simulink model "Aries_2"  (R2026a)
settings: Solver=VariableStepAuto  StopTime=0.05
undefined symbols (not defined in the file): physconst
libraries: phasedtxrxlib x4, phasedenvlib x3, phaseddetectlib x2, phasedwavlib x1, phasedbflib x1
settings Model: Creator=Anunnya  LastModifiedBy=Anunnya

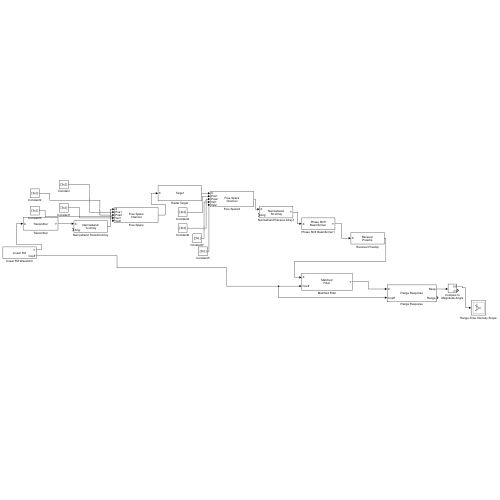
[thumbnail: Simulink's stored preview of the top-level diagram]
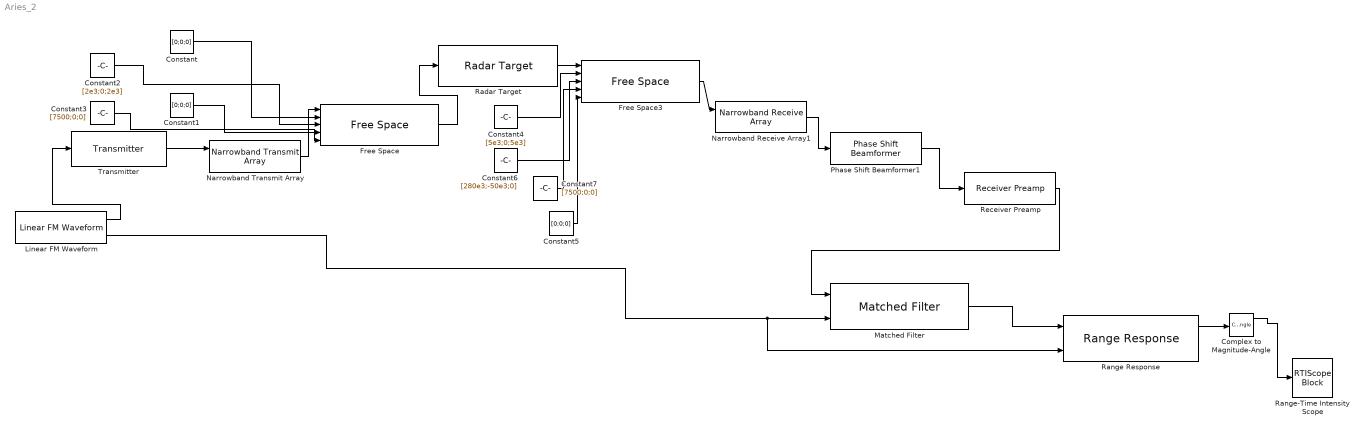
== system Aries_2 ==
  Complex to Magnitude-Angle : ComplexToMagnitudeAngle
  Constant : Constant  Value=[0;0;0]
  Constant1 : Constant  Value=[0;0;0]
  Constant2 : Constant  Value=[2e3;0;2e3]
  Constant3 : Constant  Value=[7500;0;0]
  Constant4 : Constant  Value=[5e3;0;5e3]
  Constant5 : Constant  Value=[0;0;0]
  Constant6 : Constant  Value=[280e3;-50e3;0]
  Constant7 : Constant  Value=[7500;0;0]
  Free Space : phasedenvlib/Free Space  PropagationSpeed=physconst( 'LightSpeed' )  OperatingFrequency=206.5e6  TwoWayPropagation=off  SampleRateFromInputCheckbox=on  SampleRate=1e6  MaximumDistanceSource=Property  MaximumDistance=10e3  MaximumNumInputSamplesSource=Auto  MaximumNumInputSamples=1000  FractionalDelayMethod=Linear  SimulateUsing=Interpreted execution
  Free Space3 : phasedenvlib/Free Space  PropagationSpeed=physconst( 'LightSpeed' )  OperatingFrequency=206.5e6  TwoWayPropagation=off  SampleRateFromInputCheckbox=on  SampleRate=1e6  MaximumDistanceSource=Property  MaximumDistance=10e3  MaximumNumInputSamplesSource=Auto  MaximumNumInputSamples=1000  FractionalDelayMethod=Linear  SimulateUsing=Interpreted execution
  Linear FM Waveform : phasedwavlib/Linear FM Waveform  SampleRate=1e6  DurationSpecification=Pulse width  PulseWidth=20e-6  DutyCycle=0.5  PRF=1000  PRFSelectionInputPort=off  SimulationTimeSource=Derive from waveform parameters  SweepBandwidth=5e6  SweepDirection=Up  SweepInterval=Positive  Envelope=Rectangular  FrequencyOffsetSource=Property  FrequencyOffset=0  OutputFormat=Pulses  NumSamples=100  NumPulses=16  PRFOutputPort=off  CoefficientsOutputPort=on  SimulateUsing=Interpreted execution
  Matched Filter : phaseddetectlib/Matched Filter  CoefficientsSource=Input port  Coefficients=[ 1; 1 ]  SpectrumWindow=None  CustomSpectrumWindow=@hamming  SpectrumRange=[ 0, 1e5 ]  SampleRateFromInputCheckbox=on  SampleRate=1e6  SidelobeAttenuation=30  Beta=0.5  Nbar=4  GainOutputPort=off  MaximumNumInputSamplesSource=Auto  MaximumNumInputSamples=100  SimulateUsing=Interpreted execution
  Narrowband Receive Array1 : phasedtxrxlib/Narrowband Receive Array  PropagationSpeed=physconst( 'LightSpeed' )  OperatingFrequency=206.5e6  Wavefront=Plane  SensorGainMeasure=dB  Polarization=None  WeightsInputPort=off  SimulateUsing=Interpreted execution  Sensor=|
      | phased.ConformalArray(ElementPosition=[ 0       0.726    0.363   -0.363   -0.726   -0.363    0.363    1.452    1.089    0.726     0    -0.726   -1.089   -1.452   -1.089   -0.726    0     0.726    1.089;
      |   0       0        0.629    0.629    0       -0.629   -0.629    0        1.258    1.887   2.516    1.887    1.258     0      -1.258   -1.887   -2.516   -1.887   -1.258;
      |   0       0        0        0        0        0        0         0        0        0        0        0        0         0       0        0        0        0        0],Element=phased.IsotropicAntennaElement())
  Narrowband Transmit Array : phasedtxrxlib/Narrowband Transmit Array  PropagationSpeed=physconst( 'LightSpeed' )  OperatingFrequency=206.5e6  CombineRadiatedSignals=on  SensorGainMeasure=dB  Polarization=None  WeightsInputPort=off  SimulateUsing=Interpreted execution  Sensor=phased.ULA(Element=phased.IsotropicAntennaElement(),NumElements=8,ElementSpacing=0.726)
  Phase Shift Beamformer1 : phasedbflib/Phase Shift Beamformer  PropagationSpeed=physconst( 'LightSpeed' )  OperatingFrequency=206.5e6  DirectionSource=Property  Direction=[ 0; 0 ]  NumPhaseShifterBits=0  WeightsNormalization=Distortionless  WeightsOutputPort=off  SimulateUsing=Interpreted execution  SensorArray=|
      | phased.ConformalArray(ElementPosition=[ 0       0.726    0.363   -0.363   -0.726   -0.363    0.363    1.452    1.089    0.726     0    -0.726   -1.089   -1.452   -1.089   -0.726    0     0.726    1.089;
      |   0       0        0.629    0.629    0       -0.629   -0.629    0        1.258    1.887   2.516    1.887    1.258     0      -1.258   -1.887   -2.516   -1.887   -1.258;
      |   0       0        0        0        0        0        0         0        0        0        0        0        0         0       0        0        0        0        0],Element=phased.IsotropicAntennaElement())
  Radar Target : phasedenvlib/Radar Target  EnablePolarization=off  Mode=Monostatic  MeanRCSSource=Property  ScatteringMatrixSource=Property  MeanRCS=1e3  ScatteringMatrix=eye( 2 )  Model=Nonfluctuating  PropagationSpeed=physconst( 'LightSpeed' )  OperatingFrequency=206.5e6  SeedSource=Auto  Seed=0  SimulateUsing=Interpreted execution
  Range Response : phaseddetectlib/Range Response  Mode=Bistatic  RangeMethod=Matched filter  PropagationSpeed=physconst( 'lightspeed' )  SampleRateFromInputCheckbox=on  SampleRate=1e6  SweepSlope=1e9  DechirpInput=off  RangeFFTLengthSource=Auto  RangeFFTLength=1024  RangeWindow=None  RangeSidelobeAttenuation=30  CustomRangeWindow=@hamming  ReferenceRangeCentered=on  ReferenceRange=0  MaximumNumInputSamplesSource=Auto  MaximumNumInputSamples=100  InputSignalLatency=0  SimulateUsing=Interpreted execution
  Range-Time Intensity Scope : RTIScopeBlock  WindowPosition=[1.000000,49.000000,1920.000000,1009.000000,]  ScopeFrameLocation=window
  Receiver Preamp : phasedtxrxlib/Receiver Preamp  Gain=15  LossFactor=0  NoiseMethod=Noise temperature  NoiseFigure=2  ReferenceTemperature=290  SampleRateFromInputCheckbox=on  SampleRate=1e6  NoisePower=0  EnableInputPort=off  PhaseNoiseInputPort=off  SeedSource=Auto  Seed=0  SimulateUsing=Interpreted execution
  Transmitter : phasedtxrxlib/Transmitter  Configuration=EIRP  InUseOutputPort=off  CoherentOnTransmit=on  PhaseNoiseOutputPort=off  SampleRate=1e6  SampleRateFromInputCheckbox=on  SimulateUsing=Interpreted execution  PeakPower=235e3  GainMethod=Linear  Gain=34  LossFactor=0  OIP3=Inf  Table=[ -25, 5, -1; -10, 20, -2; 0, 27, 12; 5, 28, 12 ]  NoiseMethod=None  NoiseFigure=0  NoiseFactor=1  NoiseTemperature=0  ReferenceTemperature=290  PhaseOffset=0  SeedSource=Auto  Seed=0
  wires:
  Transmitter/1 -> Narrowband Transmit Array/1
  Narrowband Transmit Array/1 -> Free Space/1
  Free Space/1 -> Radar Target/1
  Receiver Preamp/1 -> Matched Filter/1
  Radar Target/1 -> Free Space3/1
  Constant/1 -> Free Space/2
  Constant1/1 -> Free Space/4
  Constant2/1 -> Free Space/3
  Constant3/1 -> Free Space/5
  Constant4/1 -> Free Space3/2
  Constant6/1 -> Free Space3/3
  Constant7/1 -> Free Space3/4
  Constant5/1 -> Free Space3/5
  Linear FM Waveform/2 -> Range Response/2, Matched Filter/2
  Linear FM Waveform/1 -> Transmitter/1
  Matched Filter/1 -> Range Response/1
  Range Response/1 -> Complex to Magnitude-Angle/1
  Complex to Magnitude-Angle/1 -> Range-Time Intensity Scope/1
  Narrowband Receive Array1/1 -> Phase Shift Beamformer1/1
  Phase Shift Beamformer1/1 -> Receiver Preamp/1
  Free Space3/1 -> Narrowband Receive Array1/1
